simulink model "Two_Attitude_Estimation_ekf"  (R2021a)
settings: Solver=FixedStepAuto  StartTime=0.0  StopTime=200  FixedStep=Ts  RelTol=1e-5
values from neighbouring files (symbols this model uses):
  accel_filter_coef = [    0.0264    0.1405    0.3331    0.3331    0.1405    0.0264]    [quad_params_ekf.m]
  g = ref_acc(3)    [ekf_measurement_jacobian.m]    (also in quad_params_ekf.m = 9.81)
  gyro_filter_den = [ 1.0000    2.2287    2.5245    1.5773    0.5410    0.0796]    [quad_params_ekf.m]
  gyro_filter_num = [ 0.2821    1.2725    2.4208    2.4208    1.2725    0.2821]    [quad_params_ekf.m]
  I = [     0.005831943165131                   0                   0 ... (first row only)    [quad_params_ekf.m]
  Kd_rates = [0.05,0.05,0.1]'    [quad_params_ekf.m]
  Kd_vel = [0.8,0.8,0.3]'    [quad_params_ekf.m]
  Ki_vel = [0.1,0.1,0.1]'    [quad_params_ekf.m]
  km = 1.2e-7    (= 1.2e-07)    [quad_params_ekf.m]
  Kp_att = [6,6,6]'    [quad_params_ekf.m]
  Kp_pos = [7,7,3]'    [quad_params_ekf.m]
  Kp_rates = [10,10,10]'    [quad_params_ekf.m]
  Kp_vel = [3,3,5]'    [quad_params_ekf.m]
  kt = 0.9e-5    (= 9e-06)    [quad_params_ekf.m]
  L = 0.2    [quad_params_ekf.m]
  m = 0.9272    [quad_params_ekf.m]
  P_init = 0.01*eye(7)    [quad_params_ekf.m]
  Q = diag([0.015,0.0150,0.0150,0.0150,0.001,0.001,0.001])    [quad_params_ekf.m]
  q_init = [1;0;0;0]    [quad_params_ekf.m]
  R = diag([0.35,0.35,0.35,0.05,0.05,0.05])    [quad_params_ekf.m]
  rate_p_max = 3.5    [quad_params_ekf.m]
  thrust_max = thrust_max_per_motor*4    (= 32)    [quad_params_ekf.m]
  thrust_max_per_motor = 8    [quad_params_ekf.m]
  tilt_max = pi/6    (= 0.523598775598)    [quad_params_ekf.m]
  TQ_max_per_motor = km*(w_max.^2)    [quad_params_ekf.m]
  Ts = 0.001    [ekf_process_jacobian.m]    (also in ekf_process_model.m; quad_params_ekf.m)
  Ts_IMU = 0.001    [quad_params_ekf.m]
  Vb_init = [0;0;0]    [quad_params_ekf.m]
  vel_xy_max = 15    [quad_params_ekf.m]
  vel_z_max = 10    [quad_params_ekf.m]
  wb_init = [0;0;0]    [quad_params_ekf.m]
  x_0 = [1 0 0 0 0 0 0]'    [quad_params_ekf.m]
  Xe_init = [0;0;0]    [quad_params_ekf.m]
undefined symbols (not defined in the file or in its folder): IMU, p, pm_0, sigbuilder_block, Vm_0, xme_0
libraries: aerolibutil x8, simulink_extras x8, sharedtransform x7, sharedutil x6, simulink x4, pid_lib x3, aerolibcommonsys x3, aerolibnavsys x2, dspstat3 x2, mspsensorlib x1, aerolibnav x1, dspmtrx3 x1
(part 1 of 4)
settings Model: Creator=Petronas-Tareq  LastModifiedBy=Petronas-Tareq
settings SolverCC: AutoInsertRateTranBlk=on  InsertRTBMode=Always

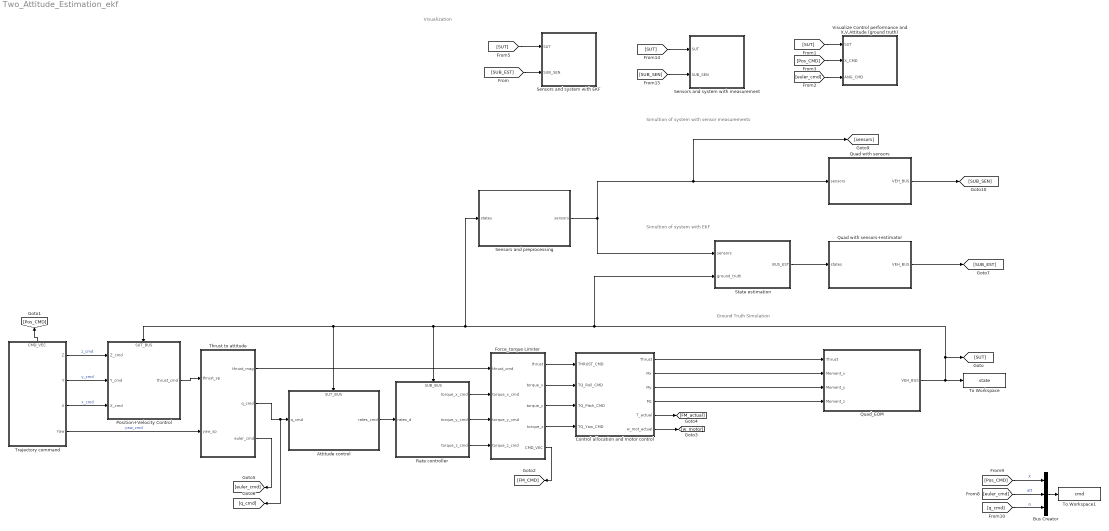
== system Two_Attitude_Estimation_ekf ==
  note: Simultion of system with sensor measurements
  note: Visualization
  note: Ground Truth Simulation
  note: Simultion of system with EKF
  Attitude control : Subsystem
      settings: PortSchema="{\"entries\":[{\"content\":{\"sides\":[{\"content\":{\"connectorIds\":[\"In1\"]},\"type\":\"ConnectorPlacement.EquallySpacedRectSide\",\"uuid\":\"19a574f6-5314-4727-8968-5b1c9712010e\"},{\"content\":{\"connectorIds\":[\"Out1\"],\"side\":\"RIGHT\"},\"type\":\"ConnectorPlacement.EquallySpacedRectSide\",\"uuid\":\"5cd6813f-6e17-48c1-918b-7c366c6d9cfa\"},{\"content\":{\"connectorIds\":[\"In2\"],\"side\":\"TOP\"},\"type\":\"ConnectorPlacement.EquallySpacedRectSide\",\"uuid\":\"b2bca67c-c4f4-4722-89a0-a16251073bfd\"}]},\"type\":\"ConnectorPlacement.EquallySpacedConnector\",\"uuid\":\"dcbf54f5-c136-40d5-a3db-9d2776e5196c\"}],\"packageUris\":[\"http://schema.mathworks.com/mf0/Connector/R2020b\"],\"version\":\"1.0\"}"
      mask Display: image('$imagefile'); % Use "Edit Image" on toolstrip to change.
  Bus Creator : BusCreator  Inputs=3
  Control allocation and motor control : Subsystem  Variant=on  VariantControlMode=label  LabelModeActiveChoice=Choice1
      mask Display: image('$imagefile'); % Use "Edit Image" on toolstrip to change.
  Force_torque Limiter : Subsystem
  Position+Velocity Control : Subsystem
      settings: PortSchema="{\"entries\":[{\"content\":{\"sides\":[{\"content\":{\"connectorIds\":[\"In1\",\"In2\",\"In3\"]},\"type\":\"ConnectorPlacement.EquallySpacedRectSide\",\"uuid\":\"cfe37ea9-b8e2-443a-9d65-596f0fda79c9\"},{\"content\":{\"connectorIds\":[\"Out1\"],\"side\":\"RIGHT\"},\"type\":\"ConnectorPlacement.EquallySpacedRectSide\",\"uuid\":\"f39f64e1-4b16-444a-b7d2-95ecb1b2a6fa\"},{\"content\":{\"connectorIds\":[\"In4\"],\"side\":\"TOP\"},\"type\":\"ConnectorPlacement.EquallySpacedRectSide\",\"uuid\":\"52402c3a-f2ac-44cf-8c94-dbfc3f851d2b\"}]},\"type\":\"ConnectorPlacement.EquallySpacedConnector\",\"uuid\":\"0122f56a-2702-493b-af7d-a25e6b9e04ed\"}],\"packageUris\":[\"http://schema.mathworks.com/mf0/Connector/R2020b\"],\"version\":\"1.0\"}"
  Quad with sensors : Subsystem
      mask Display: image('$imagefile'); % Use "Edit Image" on toolstrip to change.
  Quad with sensors+estimator : Subsystem
      mask Display: image('$imagefile'); % Use "Edit Image" on toolstrip to change.
  Quad_EOM : Subsystem
      mask Display: image('$imagefile'); % Use "Edit Image" on toolstrip to change.
  Rate controller : Subsystem
      settings: PortSchema="{\"entries\":[{\"content\":{\"sides\":[{\"content\":{\"connectorIds\":[\"In1\"]},\"type\":\"ConnectorPlacement.EquallySpacedRectSide\",\"uuid\":\"0af60e35-7b10-4750-a6af-1a3d920b4771\"},{\"content\":{\"connectorIds\":[\"Out1\",\"Out2\",\"Out3\"],\"side\":\"RIGHT\"},\"type\":\"ConnectorPlacement.EquallySpacedRectSide\",\"uuid\":\"931b0f34-b3f1-4a41-949f-3d763eca3151\"},{\"content\":{\"connectorIds\":[\"In2\"],\"side\":\"TOP\"},\"type\":\"ConnectorPlacement.EquallySpacedRectSide\",\"uuid\":\"84fe42fa-07d1-4fd9-ad2f-8c6651eaa98c\"}]},\"type\":\"ConnectorPlacement.EquallySpacedConnector\",\"uuid\":\"f603d2ac-5c20-4a82-ba8b-1c7971d6778a\"}],\"packageUris\":[\"http://schema.mathworks.com/mf0/Connector/R2020b\"],\"version\":\"1.0\"}"
  Sensors and preprocessing : Subsystem
  Sensors and system with EKF : Subsystem
  Sensors and system with measurement : Subsystem
  State estimation : Subsystem
  Thrust to attitude : Subsystem
  To Workspace : ToWorkspace  VariableName=state  SaveFormat=Timeseries  SampleTime=-1
  To Workspace1 : ToWorkspace  VariableName=cmd  SaveFormat=Timeseries  SampleTime=-1
  Trajectory command : Subsystem  Variant=on  VariantControlMode=label  LabelModeActiveChoice=5
      settings: PortSchema="{\"entries\":[{\"content\":{\"sides\":[{\"content\":{\"connectorIds\":[]},\"type\":\"ConnectorPlacement.EquallySpacedRectSide\",\"uuid\":\"8b658e99-682c-4d99-9859-63a6cdcf875c\"},{\"content\":{\"connectorIds\":[\"Out1\",\"Out2\",\"Out3\",\"Out4\"],\"side\":\"RIGHT\"},\"type\":\"ConnectorPlacement.EquallySpacedRectSide\",\"uuid\":\"566e7e32-52b1-45cc-9bb3-5343461c1cc0\"},{\"content\":{\"connectorIds\":[\"Out5\"],\"side\":\"TOP\"},\"type\":\"ConnectorPlacement.EquallySpacedRectSide\",\"uuid\":\"4cb1ab19-6483-4408-b5f4-106b35038f17\"}]},\"type\":\"ConnectorPlacement.EquallySpacedConnector\",\"uuid\":\"dc7c82fc-432d-4c18-9829-e6c2b483f5a7\"}],\"packageUris\":[\"http://schema.mathworks.com/mf0/Connector/R2020b\"],\"version\":\"1.0\"}"
  Visualize Control performance and X,V,Attitude (ground truth) : Subsystem
  wires:
  Force_torque Limiter/5(CMD_VEC) -> [FM_CMD]
  Trajectory command/2(Y) -> Position+Velocity Control/2(Y_cmd)  "y_cmd"
  Trajectory command/3(X) -> Position+Velocity Control/3(X_cmd)  "x_cmd"
  Control allocation and motor control/1(Thrust) -> Quad_EOM/1(Thrust)
  Control allocation and motor control/2(Mx) -> Quad_EOM/2(Moment_x)
  Control allocation and motor control/3(My) -> Quad_EOM/3(Moment_y)
  Control allocation and motor control/4(Mz) -> Quad_EOM/4(Moment_z)
  Control allocation and motor control/5(T_actual) -> [FM_actual]
  Control allocation and motor control/6(w_mot_actual) -> [w_motor]
  Trajectory command/1(Z) -> Position+Velocity Control/1(Z_cmd)  "z_cmd"
  Force_torque Limiter/4(torque_z) -> Control allocation and motor control/4(TQ_Yaw_CMD)
  Force_torque Limiter/3(torque_y) -> Control allocation and motor control/3(TQ_Pitch_CMD)
  Force_torque Limiter/2(torque_x) -> Control allocation and motor control/2(TQ_Roll_CMD)
  Force_torque Limiter/1(thrust) -> Control allocation and motor control/1(THRUST_CMD)
  Thrust to attitude/1(thrust_mag) -> Force_torque Limiter/1(thrust_cmd)
  Rate controller/2(torque_y_cmd) -> Force_torque Limiter/3(torque_y_cmd)
  Rate controller/3(torque_z_cmd) -> Force_torque Limiter/4(torque_z_cmd)
  Rate controller/1(torque_x_cmd) -> Force_torque Limiter/2(torque_x_cmd)
  Attitude control/1(rates_cmd) -> Rate controller/1(rates_d)
  Trajectory command/5(CMD_VEC) -> [Pos_CMD]
  Bus Creator/1 -> To Workspace1/1
  [Pos_CMD] -> Bus Creator/1  "X"
  [euler_cmd] -> Bus Creator/2  "att"
  [q_cmd] -> Bus Creator/3  "q"
  Thrust to attitude/2(q_cmd) -> Attitude control/1(q_cmd), [q_cmd]
  Thrust to attitude/3(euler_cmd) -> [euler_cmd]
  Trajectory command/4(Yaw) -> Thrust to attitude/2(yaw_sp)  "yaw_cmd"
  Position+Velocity Control/1(thrust_cmd) -> Thrust to attitude/1(thrust_sp)
  Quad_EOM/1(VEH_BUS) -> Sensors and preprocessing/1(states), Position+Velocity Control/4(SUT_BUS), Attitude control/2(SUT_BUS), Rate controller/2(SUB_BUS), State estimation/2(ground_truth), [SUT], To Workspace/1
  Sensors and preprocessing/1(sensors) -> Quad with sensors/1(sensors), [sensors], State estimation/1(sensors)
  Quad with sensors/1(VEH_BUS) -> [SUB_SEN]
  [SUB_SEN] -> Sensors and system with measurement/2(SUB_SEN)
  [SUT] -> Visualize Control performance and X,V,Attitude (ground truth)/1(SUT)
  [euler_cmd] -> Visualize Control performance and X,V,Attitude (ground truth)/3(ANG_CMD)
  [Pos_CMD] -> Visualize Control performance and X,V,Attitude (ground truth)/2(X_CMD)
  [SUT] -> Sensors and system with measurement/1(SUT)
  Quad with sensors+estimator/1(VEH_BUS) -> [SUB_EST]
  State estimation/1(BUS_EST) -> Quad with sensors+estimator/1(states)
  [SUT] -> Sensors and system with EKF/1(SUT)
  [SUB_EST] -> Sensors and system with EKF/2(SUB_SEN)

== system Two_Attitude_Estimation_ekf/Attitude control ==
  note: Attitude control (full attitude control, i.e. yaw+thrust)
  note: Attitude Error Calculation
  q_cmd : Inport
  SUT_BUS : Inport  Port=2
  Bus Selector3 : BusSelector  OutputSignals=q
  K_attitude : Gain  Gain=Kp_att
  MATLAB Function1 : MATLAB Function  TreatAsAtomicUnit=on
  Product : Product
  Quaternion Inverse : aerolibutil/Quaternion Inverse
  Quaternion multiply : aerolibutil/Quaternion Multiplication
  Selector1 : Selector  InputPortWidth=4  IndexOptions=Index vector (dialog)  Indices=1  OutputSizes=1
  Selector2 : Selector  InputPortWidth=4  IndexOptions=Index vector (dialog)  Indices=2:4  OutputSizes=1
  k : Gain  Gain=2
  rates_cmd : Outport  VectorParamsAs1DForOutWhenUnconnected=off
  wires:
  SUT_BUS/1 -> [SUT]
  q_cmd/1 -> Quaternion multiply/2  "q_d"
  [SUT] -> Bus Selector3/1
  Bus Selector3/1 -> Quaternion Inverse/1  "<q>"
  Product/1 -> k/1  "error"
  Selector1/1 -> MATLAB Function1/1(q0)  "q0"
  MATLAB Function1/1(y) -> Product/1
  Selector2/1 -> Product/2  "q_vec"
  Quaternion multiply/1 -> Selector2/1, Selector1/1  "qe"
  k/1 -> K_attitude/1
  Quaternion Inverse/1 -> Quaternion multiply/1
  K_attitude/1 -> rates_cmd/1  "rates_cmd"

== system Two_Attitude_Estimation_ekf/Control allocation and motor control ==
  note: 1) Add Subsystem or Model blocks as valid variant choices.
      | 2) You cannot connect blocks at this level. At simulation, connectivity is automatically
      | determined, based on the active variant and port name matching.
  THRUST_CMD : Inport
  TQ_Roll_CMD : Inport  Port=2
  TQ_Pitch_CMD : Inport  Port=3
  TQ_Yaw_CMD : Inport  Port=4
  Ideal Actuators with allocation : Subsystem  VariantControl=Choice2
  Ideal Actuattion (direct transfer) : Subsystem  VariantControl=Choice1
  Thrust : Outport
  Mx : Outport  Port=2
  My : Outport  Port=3
  Mz : Outport  Port=4
  T_actual : Outport  Port=5
  w_mot_actual : Outport  Port=6

== system Two_Attitude_Estimation_ekf/Force_torque Limiter ==
  thrust_cmd : Inport
  torque_x_cmd : Inport  Port=2
  torque_y_cmd : Inport  Port=3
  torque_z_cmd : Inport  Port=4
  Mux : Mux
  Saturation : Saturate  UpperLimit=thrust_max  LowerLimit=-thrust_max
      settings: AttributesFormatString=|
      | MAX =    %<UpperLimit>
      | MIN = %<LowerLimit>
  Saturation1 : Saturate  UpperLimit=2*TQ_max_per_motor  LowerLimit=-2*TQ_max_per_motor
      settings: AttributesFormatString=|
      | MAX =    %<UpperLimit>
      | MIN = %<LowerLimit>
  Saturation2 : Saturate  UpperLimit=thrust_max_per_motor*L  LowerLimit=-thrust_max_per_motor *L
      settings: AttributesFormatString=|
      | MAX =    %<UpperLimit>
      | MIN = %<LowerLimit>
  Saturation3 : Saturate  UpperLimit=thrust_max_per_motor*L  LowerLimit=-thrust_max_per_motor *L
      settings: AttributesFormatString=|
      | MAX =    %<UpperLimit>
      | MIN = %<LowerLimit>
  Scope : Scope
  thrust : Outport  VectorParamsAs1DForOutWhenUnconnected=off
  torque_x : Outport  Port=2  VectorParamsAs1DForOutWhenUnconnected=off
  torque_y : Outport  Port=3  VectorParamsAs1DForOutWhenUnconnected=off
  torque_z : Outport  Port=4  VectorParamsAs1DForOutWhenUnconnected=off
  CMD_VEC : Outport  Port=5  VectorParamsAs1DForOutWhenUnconnected=off
  wires:
  torque_z_cmd/1 -> Saturation1/1
  thrust_cmd/1 -> Saturation/1
  torque_y_cmd/1 -> Saturation2/1
  torque_x_cmd/1 -> Saturation3/1
  Saturation/1 -> [THRUST], thrust/1
  Saturation3/1 -> [TQ_Roll_X], torque_x/1
  Saturation2/1 -> [TQ_Pitch_Y], torque_y/1
  Saturation1/1 -> [TQ_Yaw_Z], torque_z/1
  Mux/1 -> Scope/1, CMD_VEC/1
  [THRUST] -> Mux/1
  [TQ_Roll_X] -> Mux/2
  [TQ_Pitch_Y] -> Mux/3
  [TQ_Yaw_Z] -> Mux/4

== system Two_Attitude_Estimation_ekf/Position+Velocity Control ==
  note: Velocity PID controller
  note: Position P controller
  Z_cmd : Inport
  Y_cmd : Inport  Port=2
  X_cmd : Inport  Port=3
  SUT_BUS : Inport  Port=4
  Bus Selector3 : BusSelector  OutputSignals=Xe,Ve
  Mux : Mux  Inputs=3
  Position P Controller : Subsystem
  To Workspace2 : ToWorkspace  VariableName=thrust_sp  SaveFormat=Timeseries  SampleTime=-1
  Velocity PID Controller : Subsystem
  acc setpoint : Constant  Value=[0;0;0]
  thrust_cmd : Outport
  wires:
  SUT_BUS/1 -> [SUT]
  [SUT] -> Bus Selector3/1
  Bus Selector3/1 -> [P]  "<Xe>"
  Mux/1 -> [P_sp]
  acc setpoint/1 -> [acc_sp]
  [acc_sp] -> Velocity PID Controller/3(acc_ff)  "acc_feedforwad"
  Position P Controller/1(V_sp) -> Velocity PID Controller/1(vel_cmd)  "vel_cmd"
  [P_sp] -> Position P Controller/1(pos_cmd)
  [P] -> Position P Controller/2(pos_cur)
  [V] -> Velocity PID Controller/2(vel_cur)
  Velocity PID Controller/1(thrust_sp) -> To Workspace2/1, thrust_cmd/1  "thrust_cmd"
  Bus Selector3/2 -> [V]  "<Ve>"
  Z_cmd/1 -> Mux/3
  X_cmd/1 -> Mux/1
  Y_cmd/1 -> Mux/2

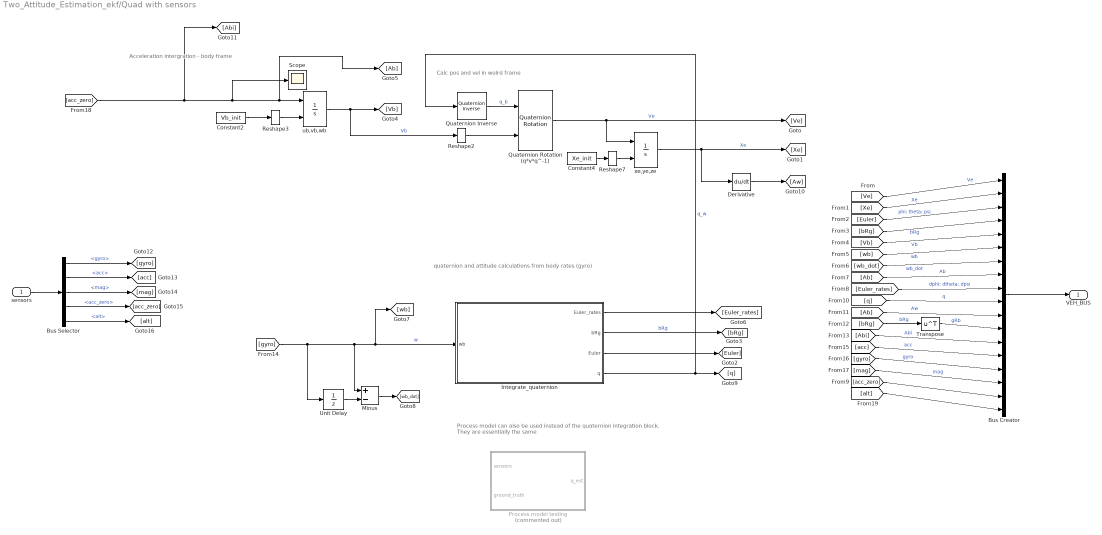
== system Two_Attitude_Estimation_ekf/Quad with sensors ==
  note: Process model can also be used instead of the
      |  quaternion integration block. They are essentially the same
  note: Acceleration intergration - body frame
  note: Calc pos and vel in wolrd frame
  note: quaternion and attitude calculations from body rates (gyro)
  sensors : Inport
  Bus Creator : BusCreator  Inputs=18
  Bus Selector : BusSelector  OutputSignals=gyro,acc,mag,acc_zero,alt
  Constant2 : Constant  Value=Vb_init  OutDataTypeStr=Inherit: Inherit via back propagation
  Constant4 : Constant  Value=Xe_init  OutDataTypeStr=Inherit: Inherit via back propagation
  Derivative : Derivative
  Integrate_quaternion : Subsystem
  Minus : Sum  Inputs=+-
  Process model testing : Subsystem  Commented=on
  Quaternion Inverse : aerolibutil/Quaternion Inverse
  Quaternion Rotation (q*v*q^-1) : aerolibutil/Quaternion Rotation
  Reshape2 : Reshape  OutputDimensionality=Column vector (2-D)
  Reshape3 : Reshape  OutputDimensionality=Column vector (2-D)
  Reshape7 : Reshape  OutputDimensionality=Column vector (2-D)
  Scope : Scope
  Transpose : Math  Operator=transpose  SaturateOnIntegerOverflow=on
  Unit Delay : UnitDelay  SampleTime=-1  HasFrameUpgradeWarning=on
  ub,vb,wb : Integrator  InitialConditionSource=external  InitialCondition=Vm_0
  xe,ye,ze : Integrator  InitialConditionSource=external  InitialCondition=xme_0
  VEH_BUS : Outport  VectorParamsAs1DForOutWhenUnconnected=off
  wires:
  [Euler] -> Bus Creator/3  "phi; theta; psi"
  [Xe] -> Bus Creator/2  "Xe"
  [Ve] -> Bus Creator/1  "Ve"
  [bRg] -> Bus Creator/4  "bRg"
  [Ab] -> Bus Creator/8  "Ab"
  [wb_dot] -> Bus Creator/7  "wb_dot"
  Bus Creator/1 -> VEH_BUS/1
  [Vb] -> Bus Creator/5  "Vb"
  [wb] -> Bus Creator/6  "wb"
  [Euler_rates] -> Bus Creator/9  "dphi; dtheta; dpsi"
  Constant2/1 -> Reshape3/1
  Integrate_quaternion/2(bRg) -> [bRg]  "bRg"
  Constant4/1 -> Reshape7/1
  Reshape3/1 -> ub,vb,wb/2
  Reshape7/1 -> xe,ye,ze/2
  Quaternion Rotation (q*v*q^-1)/1 -> xe,ye,ze/1, [Ve]  "Ve"
  xe,ye,ze/1 -> Derivative/1, [Xe]  "Xe"
  [gyro] -> Unit Delay/1, Minus/1, Integrate_quaternion/1(wb), [wb]  "w"
  ub,vb,wb/1 -> [Vb], Reshape2/1  "Vb"
  Integrate_quaternion/1(Euler_rates) -> [Euler_rates]
  Integrate_quaternion/3(Euler) -> [Euler]
  [q] -> Bus Creator/10  "q"
  Integrate_quaternion/4(q) -> Quaternion Inverse/1, [q]  "q_w"
  Reshape2/1 -> Quaternion Rotation (q*v*q^-1)/2
  Quaternion Inverse/1 -> Quaternion Rotation (q*v*q^-1)/1  "q_b"
  Derivative/1 -> [Aw]
  [Ab] -> Bus Creator/11  "Aw"
  [bRg] -> Transpose/1  "bRg"
  Transpose/1 -> Bus Creator/12  "gRb"
  [Abi] -> Bus Creator/13  "Abi"
  Unit Delay/1 -> Minus/2
  Minus/1 -> [wb_dot]
  Bus Selector/1 -> [gyro]  "<gyro>"
  Bus Selector/2 -> [acc]  "<acc>"
  sensors/1 -> Bus Selector/1
  [acc_zero] -> [Abi], Scope/1, [Ab], ub,vb,wb/1
  [acc] -> Bus Creator/14  "acc"
  [gyro] -> Bus Creator/15  "gyro"
  Bus Selector/3 -> [mag]  "<mag>"
  [mag] -> Bus Creator/16  "mag"
  Bus Selector/4 -> [acc_zero]  "<acc_zero>"
  [acc_zero] -> Bus Creator/17
  Bus Selector/5 -> [alt]  "<alt>"
  [alt] -> Bus Creator/18

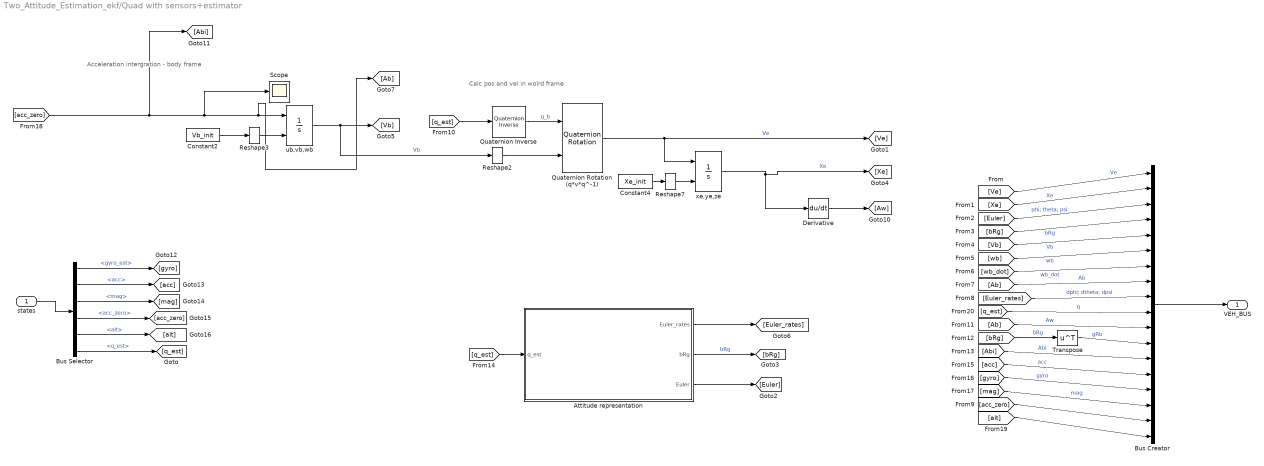
== system Two_Attitude_Estimation_ekf/Quad with sensors+estimator ==
  note: Calc pos and vel in wolrd frame
  note: Acceleration intergration - body frame
  states : Inport
  Attitude representation : Subsystem
  Bus Creator : BusCreator  Inputs=18
  Bus Selector : BusSelector  OutputSignals=gyro_est,acc,mag,acc_zero,alt,q_est
  Constant2 : Constant  Value=Vb_init  OutDataTypeStr=Inherit: Inherit via back propagation
  Constant4 : Constant  Value=Xe_init  OutDataTypeStr=Inherit: Inherit via back propagation
  Derivative : Derivative
  Quaternion Inverse : aerolibutil/Quaternion Inverse
  Quaternion Rotation (q*v*q^-1) : aerolibutil/Quaternion Rotation
  Reshape2 : Reshape  OutputDimensionality=Column vector (2-D)
  Reshape3 : Reshape  OutputDimensionality=Column vector (2-D)
  Reshape7 : Reshape  OutputDimensionality=Column vector (2-D)
  Scope : Scope
  Transpose : Math  Operator=transpose  SaturateOnIntegerOverflow=on
  ub,vb,wb : Integrator  InitialConditionSource=external  InitialCondition=Vm_0
  xe,ye,ze : Integrator  InitialConditionSource=external  InitialCondition=xme_0
  VEH_BUS : Outport  VectorParamsAs1DForOutWhenUnconnected=off
  wires:
  [Euler] -> Bus Creator/3  "phi; theta; psi"
  [Xe] -> Bus Creator/2  "Xe"
  [Ve] -> Bus Creator/1  "Ve"
  [bRg] -> Bus Creator/4  "bRg"
  [Ab] -> Bus Creator/8  "Ab"
  [wb_dot] -> Bus Creator/7  "wb_dot"
  Bus Creator/1 -> VEH_BUS/1
  [Vb] -> Bus Creator/5  "Vb"
  [wb] -> Bus Creator/6  "wb"
  [Euler_rates] -> Bus Creator/9  "dphi; dtheta; dpsi"
  Attitude representation/2(bRg) -> [bRg]  "bRg"
  Attitude representation/1(Euler_rates) -> [Euler_rates]
  Attitude representation/3(Euler) -> [Euler]
  [q_est] -> Bus Creator/10  "q"
  [Ab] -> Bus Creator/11  "Aw"
  [bRg] -> Transpose/1  "bRg"
  Transpose/1 -> Bus Creator/12  "gRb"
  [Abi] -> Bus Creator/13  "Abi"
  Bus Selector/1 -> [gyro]  "<gyro_est>"
  Bus Selector/2 -> [acc]  "<acc>"
  states/1 -> Bus Selector/1
  [acc] -> Bus Creator/14  "acc"
  [gyro] -> Bus Creator/15  "gyro"
  Bus Selector/3 -> [mag]  "<mag>"
  [mag] -> Bus Creator/16  "mag"
  Bus Selector/4 -> [acc_zero]  "<acc_zero>"
  [acc_zero] -> Bus Creator/17
  [alt] -> Bus Creator/18
  [q_est] -> Attitude representation/1(q_est)
  Bus Selector/5 -> [alt]  "<alt>"
  Bus Selector/6 -> [q_est]  "<q_est>"
  Quaternion Rotation (q*v*q^-1)/1 -> xe,ye,ze/1, [Ve]  "Ve"
  [acc_zero] -> [Abi], Scope/1, [Ab], ub,vb,wb/1
  ub,vb,wb/1 -> [Vb], Reshape2/1  "Vb"
  Constant4/1 -> Reshape7/1
  Derivative/1 -> [Aw]
  xe,ye,ze/1 -> Derivative/1, [Xe]  "Xe"
  Reshape2/1 -> Quaternion Rotation (q*v*q^-1)/2
  Reshape7/1 -> xe,ye,ze/2
  Reshape3/1 -> ub,vb,wb/2
  Quaternion Inverse/1 -> Quaternion Rotation (q*v*q^-1)/1  "q_b"
  Constant2/1 -> Reshape3/1
  [q_est] -> Quaternion Inverse/1

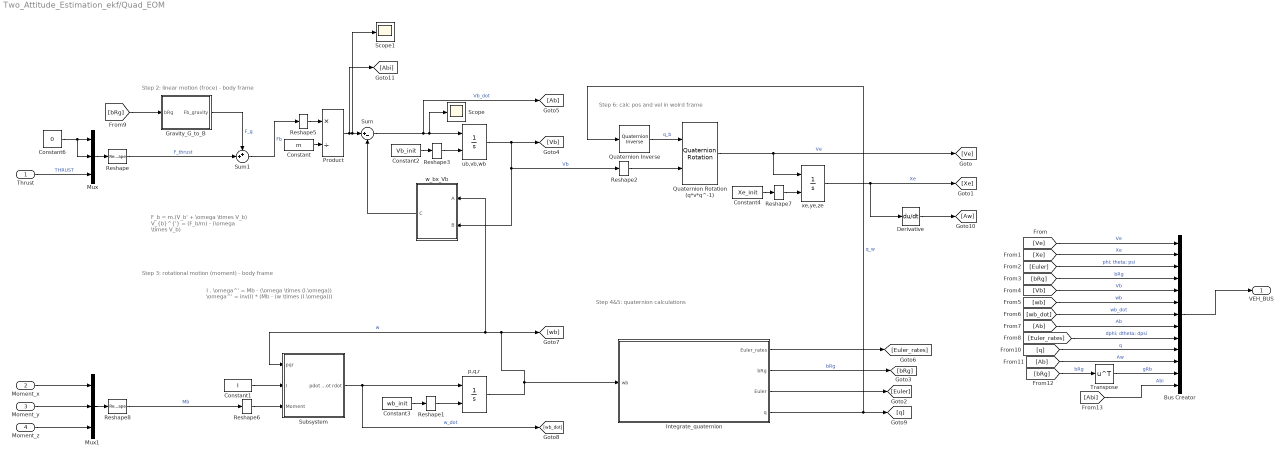
== system Two_Attitude_Estimation_ekf/Quad_EOM ==
  note: Step 3: rotational motion (moment) - body frame
  note: F_b = m.(V_b' + \omega \times V_b)
      |
      | V_{b}^{'} = (F_b/m) - (\omega \times V_b)
  note: Step 2: linear motion (froce) - body frame
  note: Step 6: calc pos and vel in wolrd frame
  note: I . \omega^' = Mb - (\omega \times (I.\omega))
      |
      | \omega^' = inv(I) * (Mb - (w \times (I.\omega)))
  note: Step 4&5: quaternion calculations
  Thrust : Inport
  Moment_x : Inport  Port=2
  Moment_y : Inport  Port=3
  Moment_z : Inport  Port=4
  Bus Creator : BusCreator  Inputs=13
  Constant : Constant  Value=m  OutDataTypeStr=Inherit: Inherit via back propagation
  Constant1 : Constant  Value=I  OutDataTypeStr=Inherit: Inherit via back propagation
  Constant2 : Constant  Value=Vb_init  OutDataTypeStr=Inherit: Inherit via back propagation
  Constant3 : Constant  Value=wb_init  OutDataTypeStr=Inherit: Inherit via back propagation
  Constant4 : Constant  Value=Xe_init  OutDataTypeStr=Inherit: Inherit via back propagation
  Constant6 : Constant  Value=0
  Derivative : Derivative
  Gravity_G_to_B : Subsystem
  Integrate_quaternion : Subsystem
  Mux : Mux  Inputs=3
  Mux1 : Mux  Inputs=3
  Product : Product  Inputs=*/  SaturateOnIntegerOverflow=on  OutDataTypeStr=Inherit: Same as first input
  Quaternion Inverse : aerolibutil/Quaternion Inverse
  Quaternion Rotation (q*v*q^-1) : aerolibutil/Quaternion Rotation
  Reshape{,1..3,5..8} (8 alike) : Reshape  OutputDimensionality=Column vector (2-D)
  Scope : Scope
  Scope1 : Scope
  Subsystem : Subsystem
  Sum : Sum  Inputs=|+-  SaturateOnIntegerOverflow=on
  Sum1 : Sum  Inputs=++|
  Transpose : Math  Operator=transpose  SaturateOnIntegerOverflow=on
  "p,q,r " : Integrator  InitialConditionSource=external  InitialCondition=pm_0
  ub,vb,wb : Integrator  InitialConditionSource=external  InitialCondition=Vm_0
  w_bx_Vb : Subsystem
      mask Display:
      | text(.5,.5,'Cross\nProduct\n\nC = AxB', ...
      | 	'HorizontalAlignment','Center',...
      | 	'VerticalAlignment','middle')
  xe,ye,ze : Integrator  InitialConditionSource=external  InitialCondition=xme_0
  VEH_BUS : Outport  VectorParamsAs1DForOutWhenUnconnected=off
  wires:
  [Euler] -> Bus Creator/3  "phi; theta; psi"
  [Xe] -> Bus Creator/2  "Xe"
  [Ve] -> Bus Creator/1  "Ve"
  [bRg] -> Bus Creator/4  "bRg"
  [Ab] -> Bus Creator/8  "Ab"
  [wb_dot] -> Bus Creator/7  "wb_dot"
  Bus Creator/1 -> VEH_BUS/1
  [Vb] -> Bus Creator/5  "Vb"
  [wb] -> Bus Creator/6  "wb"
  [Euler_rates] -> Bus Creator/9  "dphi; dtheta; dpsi"
  Reshape8/1 -> Reshape6/1  "Mb"
  Reshape6/1 -> Subsystem/3(Moment)
  Reshape1/1 -> "p,q,r "/2
  Constant2/1 -> Reshape3/1
  Subsystem/1(pdot qdot rdot) -> [wb_dot], "p,q,r "/1  "w_dot"
  Constant/1 -> Product/2
  Constant1/1 -> Subsystem/2(I)
  w_bx_Vb/1(C) -> Sum/2
  Integrate_quaternion/2(bRg) -> [bRg]  "bRg"
  Sum/1 -> [Ab], Scope/1, ub,vb,wb/1  "Vb_dot"
  Constant4/1 -> Reshape7/1
  Reshape3/1 -> ub,vb,wb/2
  Reshape7/1 -> xe,ye,ze/2
  Quaternion Rotation (q*v*q^-1)/1 -> xe,ye,ze/1, [Ve]  "Ve"
  Reshape5/1 -> Product/1
  xe,ye,ze/1 -> Derivative/1, [Xe]  "Xe"
  Sum1/1 -> Reshape5/1  "Fb"
  Constant3/1 -> Reshape1/1
  Product/1 -> [Abi], Scope1/1, Sum/1
  Constant6/1 -> Mux/2, Mux/1
  Gravity_G_to_B/1(Fb_gravity) -> Sum1/1  "F_g"
  Mux/1 -> Reshape/1
  Reshape/1 -> Sum1/2  "F_thrust"
  Thrust/1 -> Mux/3  "THRUST"
  [bRg] -> Gravity_G_to_B/1(bRg)
  Moment_y/1 -> Mux1/2
  Moment_z/1 -> Mux1/3
  Mux1/1 -> Reshape8/1
  Moment_x/1 -> Mux1/1
  "p,q,r "/1 -> [wb], Subsystem/1(pqr), w_bx_Vb/1(A), Integrate_quaternion/1(wb)  "w"
  ub,vb,wb/1 -> [Vb], Reshape2/1, w_bx_Vb/2(B)  "Vb"
  Integrate_quaternion/1(Euler_rates) -> [Euler_rates]
  Integrate_quaternion/3(Euler) -> [Euler]
  [q] -> Bus Creator/10  "q"
  Integrate_quaternion/4(q) -> Quaternion Inverse/1, [q]  "q_w"
  Reshape2/1 -> Quaternion Rotation (q*v*q^-1)/2
  Quaternion Inverse/1 -> Quaternion Rotation (q*v*q^-1)/1  "q_b"
  Derivative/1 -> [Aw]
  [Ab] -> Bus Creator/11  "Aw"
  [bRg] -> Transpose/1  "bRg"
  Transpose/1 -> Bus Creator/12  "gRb"
  [Abi] -> Bus Creator/13  "Abi"

== system Two_Attitude_Estimation_ekf/Rate controller ==
  note: Rate controller
  rates_d : Inport
  SUB_BUS : Inport  Port=2
  Bus Selector1 : BusSelector  OutputSignals=wb,wb_dot
  Demux : Demux  Outputs=3
  Kd_rates : Gain  Gain=Kd_rates
  Kp_rates : Gain  Gain=Kp_rates
  Scope : Scope  NumInputPorts=2
  Sum : Sum  Inputs=|+-
  Sum1 : Sum  Inputs=|+-
  limit rate p : Saturate  UpperLimit=rate_p_max  LowerLimit=-rate_p_max
  limit rate q : Saturate  UpperLimit=rate_p_max  LowerLimit=-rate_p_max
  limit rate r : Saturate  UpperLimit=rate_p_max  LowerLimit=-rate_p_max
  torque_x_cmd : Outport
  torque_y_cmd : Outport  Port=2
  torque_z_cmd : Outport  Port=3
  wires:
  Bus Selector1/2 -> Kd_rates/1  "<wb_dot>"
  Bus Selector1/1 -> Sum1/2, Scope/2  "<wb>"
  Demux/1 -> limit rate p/1
  Demux/2 -> limit rate q/1
  Demux/3 -> limit rate r/1
  SUB_BUS/1 -> Bus Selector1/1  "measurements"
  rates_d/1 -> Sum1/1, Scope/1
  Kd_rates/1 -> Sum/2  "w_d"
  Kp_rates/1 -> Sum/1
  Sum/1 -> Demux/1  "torques"
  Sum1/1 -> Kp_rates/1
  limit rate p/1 -> torque_x_cmd/1
  limit rate q/1 -> torque_y_cmd/1
  limit rate r/1 -> torque_z_cmd/1

== system Two_Attitude_Estimation_ekf/Sensors and preprocessing ==
  states : Inport
  Bus Creator4 : BusCreator  Inputs=5
  IMU+altitude : Subsystem
  Memory1 : Memory  InheritSampleTime=on
  Preprocessing and Filtering : Subsystem
  Scope : Scope
  Scope1 : Scope
  sensors : Outport
  wires:
  states/1 -> Memory1/1
  Bus Creator4/1 -> sensors/1
  IMU+altitude/1(acc) -> Scope/1, Preprocessing and Filtering/1(acc_raw)  "acc_raw"
  IMU+altitude/2(gyro) -> Scope1/1, Preprocessing and Filtering/2(gyro_raw)  "gyro_raw"
  Memory1/1 -> IMU+altitude/1(States)
  IMU+altitude/3(alt) -> Preprocessing and Filtering/3(alt_raw)  "alt_raw"
  IMU+altitude/4(mag) -> Preprocessing and Filtering/4(mag_raw)  "mag_raw"
  Preprocessing and Filtering/1(acc_zero) -> Bus Creator4/1  "acc_zero"
  Preprocessing and Filtering/2(acc) -> Bus Creator4/2  "acc"
  Preprocessing and Filtering/3(gyro) -> Bus Creator4/3  "gyro"
  Preprocessing and Filtering/4(alt) -> Bus Creator4/4  "alt"
  Preprocessing and Filtering/5(mag) -> Bus Creator4/5  "mag"

== system Two_Attitude_Estimation_ekf/Sensors and system with EKF ==
  note: Confirm sensors are simulated properly
  SUT : Inport
  SUB_SEN : Inport  Port=2
  "Attitude " : Scope  NumInputPorts=3
  Bus Selector : BusSelector  OutputSignals=wb
  Bus Selector1 : BusSelector  OutputSignals=phi; theta; psi
  Bus Selector2 : BusSelector  OutputSignals=Xe
  Bus Selector21 : BusSelector  OutputSignals=Xe
  Bus Selector3 : BusSelector  OutputSignals=Abi
  Bus Selector4 : BusSelector  OutputSignals=gyro
  Bus Selector5 : BusSelector  OutputSignals=acc_zero
  Bus Selector8 : BusSelector  OutputSignals=phi; theta; psi
  Demux{1..2,9,11} (4 alike) : Demux  Outputs=3
  Mux{,1..2,4..6} (6 alike) : Mux  Inputs=2
  Position : Scope  NumInputPorts=3
  Scope : Scope  NumInputPorts=2
  Scope1 : Scope  NumInputPorts=2
  wires:
  Mux4/1 -> Position/1
  Demux11/2 -> Mux5/1  "y"
  [SUT] -> Bus Selector21/1
  Demux11/1 -> Mux4/1  "x"
  Mux5/1 -> Position/2
  Demux11/3 -> Mux6/1  "z"
  Bus Selector21/1 -> Demux11/1  "<Xe>"
  [SUT] -> Bus Selector8/1
  Mux6/1 -> Position/3
  Bus Selector8/1 -> Demux9/1  "<phi; theta; psi>"
  Mux2/1 -> "Attitude "/3
  Demux9/2 -> Mux1/1  "pitch"
  Demux9/3 -> Mux2/1  "yaw"
  Mux1/1 -> "Attitude "/2
  Mux/1 -> "Attitude "/1
  Demux9/1 -> Mux/1  "roll"
  SUT/1 -> [SUT]
  SUB_SEN/1 -> [SUB_SEN]
  [SUB_SEN] -> Bus Selector1/1
  Bus Selector1/1 -> Demux1/1  "<phi; theta; psi>"
  Demux1/1 -> Mux/2  "roll_est"
  Demux1/2 -> Mux1/2  "pitch_est"
  Demux1/3 -> Mux2/2  "yaw_est"
  [SUB_SEN] -> Bus Selector2/1
  Bus Selector2/1 -> Demux2/1  "<Xe>"
  Demux2/1 -> Mux4/2  "x_est"
  Demux2/2 -> Mux5/2  "y_est"
  Demux2/3 -> Mux6/2  "z_est"
  Bus Selector/1 -> Scope/2  "<wb>"
  Bus Selector4/1 -> Scope/1  "<gyro>"
  Bus Selector5/1 -> Scope1/1  "<acc_zero>"
  [SUT] -> Bus Selector3/1
  [SUB_SEN] -> Bus Selector4/1
  [SUB_SEN] -> Bus Selector5/1
  [SUT] -> Bus Selector/1
  Bus Selector3/1 -> Scope1/2  "<Abi>"

== system Two_Attitude_Estimation_ekf/Sensors and system with measurement ==
  note: Confirm sensors are simulated properly
  SUT : Inport
  SUB_SEN : Inport  Port=2
  "Attitude " : Scope  NumInputPorts=3
  Bus Selector : BusSelector  OutputSignals=wb
  Bus Selector1 : BusSelector  OutputSignals=phi; theta; psi
  Bus Selector2 : BusSelector  OutputSignals=Xe
  Bus Selector21 : BusSelector  OutputSignals=Xe
  Bus Selector3 : BusSelector  OutputSignals=Abi
  Bus Selector4 : BusSelector  OutputSignals=gyro
  Bus Selector5 : BusSelector  OutputSignals=acc_zero
  Bus Selector8 : BusSelector  OutputSignals=phi; theta; psi
  Demux{1..2,9,11} (4 alike) : Demux  Outputs=3
  Mux{,1..2,4..6} (6 alike) : Mux  Inputs=2
  Position : Scope  NumInputPorts=3
  Scope : Scope  NumInputPorts=2
  Scope1 : Scope  NumInputPorts=2
  wires:
  Mux4/1 -> Position/1
  Demux11/2 -> Mux5/1  "y"
  [SUT] -> Bus Selector21/1
  Demux11/1 -> Mux4/1  "x"
  Mux5/1 -> Position/2
  Demux11/3 -> Mux6/1  "z"
  Bus Selector21/1 -> Demux11/1  "<Xe>"
  [SUT] -> Bus Selector8/1
  Mux6/1 -> Position/3
  Bus Selector8/1 -> Demux9/1  "<phi; theta; psi>"
  Mux2/1 -> "Attitude "/3
  Demux9/2 -> Mux1/1  "pitch"
  Demux9/3 -> Mux2/1  "yaw"
  Mux1/1 -> "Attitude "/2
  Mux/1 -> "Attitude "/1
  Demux9/1 -> Mux/1  "roll"
  SUT/1 -> [SUT]
  SUB_SEN/1 -> [SUB_SEN]
  [SUB_SEN] -> Bus Selector1/1
  Bus Selector1/1 -> Demux1/1  "<phi; theta; psi>"
  Demux1/1 -> Mux/2  "roll_est"
  Demux1/2 -> Mux1/2  "pitch_est"
  Demux1/3 -> Mux2/2  "yaw_est"
  [SUB_SEN] -> Bus Selector2/1
  Bus Selector2/1 -> Demux2/1  "<Xe>"
  Demux2/1 -> Mux4/2  "x_est"
  Demux2/2 -> Mux5/2  "y_est"
  Demux2/3 -> Mux6/2  "z_est"
  Bus Selector/1 -> Scope/2  "<wb>"
  Bus Selector4/1 -> Scope/1  "<gyro>"
  Bus Selector5/1 -> Scope1/1  "<acc_zero>"
  [SUT] -> Bus Selector3/1
  [SUB_SEN] -> Bus Selector4/1
  [SUB_SEN] -> Bus Selector5/1
  [SUT] -> Bus Selector/1
  Bus Selector3/1 -> Scope1/2  "<Abi>"

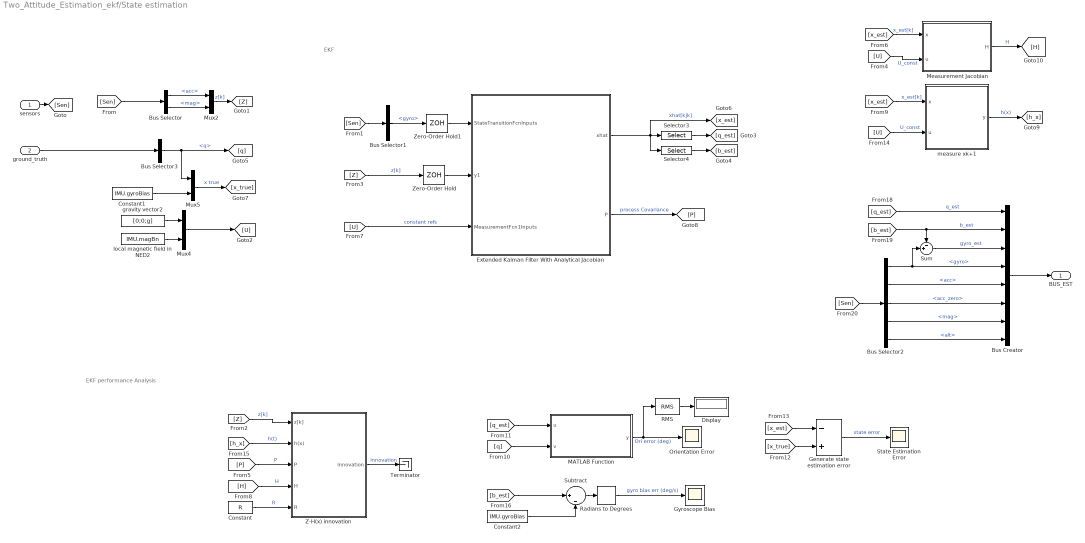
== system Two_Attitude_Estimation_ekf/State estimation ==
  note: EKF
  note: EKF performance Analysis
  sensors : Inport
  ground_truth : Inport  Port=2
  Bus Creator : BusCreator  Inputs=8
  Bus Selector : BusSelector  OutputSignals=acc,mag
  Bus Selector1 : BusSelector  OutputSignals=gyro
  Bus Selector2 : BusSelector  OutputSignals=gyro,acc,acc_zero,mag,alt
  Bus Selector3 : BusSelector  OutputSignals=q
  Constant : Constant  Value=R
  Constant1 : Constant  Value=IMU.gyroBias
  Constant2 : Constant  Value=IMU.gyroBias
  Display : Display
  Extended Kalman Filter With Analytical Jacobian : Subsystem  AncestorBlock=sharedTrackingLibrary/Extended Kalman Filter  mask(Extended Kalman Filter){StateTransitionFcn=ekf_process_model, HasStateTransitionJacobianFcn=on, StateTransitionJacobianFcn=ekf_process_jacobian, HasAdditiveProcessNoise=Additive, ProcessNoise=Q, HasTimeVaryingProcessNoise=off, HasStateTransitionFcnExtraArgument=1, InitialState=x_0, InitialStateCovariance=P_init, MeasurementFcn1=ekf_measurement_model, HasMeasurementJacobianFcn1=on, MeasurementJacobianFcn1=ekf_measurement_jacobian, HasMeasurementEnablePort1=off, HasAdditiveMeasurementNoise1=Additive, MeasurementNoise1=R, HasTimeVaryingMeasurementNoise1=off, HasMeasurementFcnExtraArgument1=1, MeasurementFcn2=myMeasurementFcn, HasMeasurementJacobianFcn2=off, MeasurementJacobianFcn2=, HasMeasurementEnablePort2=off, HasAdditiveMeasurementNoise2=Additive, MeasurementNoise2=1, HasTimeVaryingMeasurementNoise2=off, HasMeasurementFcnExtraArgument2=0, MeasurementFcn3=myMeasurementFcn, HasMeasurementJacobianFcn3=off, MeasurementJacobianFcn3=, HasMeasurementEnablePort3=off, HasAdditiveMeasurementNoise3=Additive, MeasurementNoise3=1, HasTimeVaryingMeasurementNoise3=off, HasMeasurementFcnExtraArgument3=0, MeasurementFcn4=myMeasurementFcn, HasMeasurementJacobianFcn4=off, MeasurementJacobianFcn4=, HasMeasurementEnablePort4=off, HasAdditiveMeasurementNoise4=Additive, MeasurementNoise4=1, HasTimeVaryingMeasurementNoise4=off, HasMeasurementFcnExtraArgument4=0, MeasurementFcn5=myMeasurementFcn, HasMeasurementJacobianFcn5=off, MeasurementJacobianFcn5=, HasMeasurementEnablePort5=off, HasAdditiveMeasurementNoise5=Additive, MeasurementNoise5=1, HasTimeVaryingMeasurementNoise5=off, HasMeasurementFcnExtraArgument5=0, EnableMultirate=off, StateTransitionFcnSampleTime=1, MeasurementFcn1SampleTime=1, MeasurementFcn2SampleTime=1, MeasurementFcn3SampleTime=1, MeasurementFcn4SampleTime=1, MeasurementFcn5SampleTime=1, UseCurrentEstimator=off, OutputStateCovariance=on, DataType=double, SampleTime=Ts, NumberOfMeasurements=1}
      mask prompts: HasStateTransitionJacobianFcn "shared_tracking:blocks:maskPromptEKFJacobian"; HasTimeVaryingProcessNoise "shared_tracking:blocks:maskPromptEKFUKFTimeVarying"; HasMeasurementJacobianFcn1 "shared_tracking:blocks:maskPromptEKFJacobian"; HasMeasurementEnablePort1 "shared_tracking:blocks:maskPromptEnablePort"; HasTimeVaryingMeasurementNoise1 "shared_tracking:blocks:maskPromptEKFUKFTimeVarying"; HasMeasurementJacobianFcn2 "shared_tracking:blocks:maskPromptEKFJacobian"; HasMeasurementEnablePort2 "shared_tracking:blocks:maskPromptEnablePort"; HasTimeVaryingMeasurementNoise2 "shared_tracking:blocks:maskPromptEKFUKFTimeVarying"; HasMeasurementJacobianFcn3 "shared_tracking:blocks:maskPromptEKFJacobian"; HasMeasurementEnablePort3 "shared_tracking:blocks:maskPromptEnablePort"; HasTimeVaryingMeasurementNoise3 "shared_tracking:blocks:maskPromptEKFUKFTimeVarying"; HasMeasurementJacobianFcn4 "shared_tracking:blocks:maskPromptEKFJacobian"; HasMeasurementEnablePort4 "shared_tracking:blocks:maskPromptEnablePort"; HasTimeVaryingMeasurementNoise4 "shared_tracking:blocks:maskPromptEKFUKFTimeVarying"; HasMeasurementJacobianFcn5 "shared_tracking:blocks:maskPromptEKFJacobian"; HasMeasurementEnablePort5 "shared_tracking:blocks:maskPromptEnablePort"; HasTimeVaryingMeasurementNoise5 "shared_tracking:blocks:maskPromptEKFUKFTimeVarying"; EnableMultirate "shared_tracking:blocks:maskPromptEnableMultirate"; StateTransitionFcnSampleTime "shared_tracking:blocks:maskPromptStateTransition"; MeasurementFcn1SampleTime "shared_tracking:blocks:maskPromptMeasurement1"; MeasurementFcn2SampleTime "shared_tracking:blocks:maskPromptMeasurement2"; MeasurementFcn3SampleTime "shared_tracking:blocks:maskPromptMeasurement3"; MeasurementFcn4SampleTime "shared_tracking:blocks:maskPromptMeasurement4"; MeasurementFcn5SampleTime "shared_tracking:blocks:maskPromptMeasurement5"; UseCurrentEstimator "shared_tracking:blocks:maskPromptUseCurrentEstimator"; OutputStateCovariance "shared_tracking:blocks:maskPromptOutputStateCovariance"; DataType "shared_tracking:blocks:maskPromptDataType"; SampleTime "shared_tracking:blocks:maskPromptSampleTime"
      mask help: shared_tracking:blocks:maskPromptEKFDescription
      mask init:
      | matlabshared.tracking.internal.blocks.maskInitializationScriptEKF
      mask Help: eval('matlabshared.tracking.internal.blocks.controlIdentLaunchDocPage(''EKF'')')
      mask Callback HasStateTransitionJacobianFcn: matlabshared.tracking.internal.blocks.dialogCallbacksEKFUKFPF(gcbh(),'checkBoxHasJacobianFcn','StateTransition');
      mask TypeOptions HasAdditiveProcessNoise: shared_tracking:blocks:maskPromptEKFUKFAdditiveNoise | shared_tracking:blocks:maskPromptEKFUKFNonAdditiveNoise
      mask Callback HasTimeVaryingProcessNoise: matlabshared.tracking.internal.blocks.dialogCallbacksEKFUKFPF(gcbh,'checkboxIsCovarianceTimeVarying','HasTimeVaryingProcessNoise','ProcessNoise')
      mask Callback HasMeasurementJacobianFcn1: matlabshared.tracking.internal.blocks.dialogCallbacksEKFUKFPF(gcbh(),'checkBoxHasJacobianFcn','Measurement','1');
      mask TypeOptions HasAdditiveMeasurementNoise1: shared_tracking:blocks:maskPromptEKFUKFAdditiveNoise | shared_tracking:blocks:maskPromptEKFUKFNonAdditiveNoise
      mask Callback HasTimeVaryingMeasurementNoise1: matlabshared.tracking.internal.blocks.dialogCallbacksEKFUKFPF(gcbh,'checkboxIsCovarianceTimeVarying','HasTimeVaryingMeasurementNoise1','MeasurementNoise1')
      mask Callback HasMeasurementJacobianFcn2: matlabshared.tracking.internal.blocks.dialogCallbacksEKFUKFPF(gcbh(),'checkBoxHasJacobianFcn','Measurement','2');
      mask TypeOptions HasAdditiveMeasurementNoise2: shared_tracking:blocks:maskPromptEKFUKFAdditiveNoise | shared_tracking:blocks:maskPromptEKFUKFNonAdditiveNoise
      mask Callback HasTimeVaryingMeasurementNoise2: matlabshared.tracking.internal.blocks.dialogCallbacksEKFUKFPF(gcbh,'checkboxIsCovarianceTimeVarying','HasTimeVaryingMeasurementNoise2','MeasurementNoise2')
      mask Callback HasMeasurementJacobianFcn3: matlabshared.tracking.internal.blocks.dialogCallbacksEKFUKFPF(gcbh(),'checkBoxHasJacobianFcn','Measurement','3');
      mask TypeOptions HasAdditiveMeasurementNoise3: shared_tracking:blocks:maskPromptEKFUKFAdditiveNoise | shared_tracking:blocks:maskPromptEKFUKFNonAdditiveNoise
      mask Callback HasTimeVaryingMeasurementNoise3: matlabshared.tracking.internal.blocks.dialogCallbacksEKFUKFPF(gcbh,'checkboxIsCovarianceTimeVarying','HasTimeVaryingMeasurementNoise3','MeasurementNoise3')
      mask Callback HasMeasurementJacobianFcn4: matlabshared.tracking.internal.blocks.dialogCallbacksEKFUKFPF(gcbh(),'checkBoxHasJacobianFcn','Measurement','4');
      mask TypeOptions HasAdditiveMeasurementNoise4: shared_tracking:blocks:maskPromptEKFUKFAdditiveNoise | shared_tracking:blocks:maskPromptEKFUKFNonAdditiveNoise
      mask Callback HasTimeVaryingMeasurementNoise4: matlabshared.tracking.internal.blocks.dialogCallbacksEKFUKFPF(gcbh,'checkboxIsCovarianceTimeVarying','HasTimeVaryingMeasurementNoise4','MeasurementNoise4')
      mask Callback HasMeasurementJacobianFcn5: matlabshared.tracking.internal.blocks.dialogCallbacksEKFUKFPF(gcbh(),'checkBoxHasJacobianFcn','Measurement','5');
      mask TypeOptions HasAdditiveMeasurementNoise5: shared_tracking:blocks:maskPromptEKFUKFAdditiveNoise | shared_tracking:blocks:maskPromptEKFUKFNonAdditiveNoise
      mask Callback HasTimeVaryingMeasurementNoise5: matlabshared.tracking.internal.blocks.dialogCallbacksEKFUKFPF(gcbh,'checkboxIsCovarianceTimeVarying','HasTimeVaryingMeasurementNoise5','MeasurementNoise5')
      mask Callback EnableMultirate: matlabshared.tracking.internal.blocks.dialogCallbacksEKFUKFPF(gcbh,'checkBoxHasMultirate')
      mask TypeOptions DataType: shared_tracking:blocks:maskPromptDouble | shared_tracking:blocks:maskPromptSingle
      mask Callback NumberOfMeasurements: matlabshared.tracking.internal.blocks.dialogCallbacksEKFUKFPF(gcbh,'editboxNumberOfMeasurements','MeasurementFcn');
      mask DialogControl DescGroupVar Prompt: shared_tracking:blocks:maskPromptEKFTitle
      mask DialogControl TabSystemModel Prompt: shared_tracking:blocks:maskPromptSystemModel
      mask DialogControl GroupStateTransition Prompt: shared_tracking:blocks:maskPromptStateTransition
      mask DialogControl StateTransitionFunctionText Prompt: shared_tracking:blocks:maskPromptFunction
      mask DialogControl HasStateTransitionJacobianFcn Prompt: Jacobian
      mask DialogControl Spacer Prompt: (Add text here)
      mask DialogControl ProcessNoiseText Prompt: shared_tracking:blocks:maskPromptEKFUKFProcessNoise
      mask DialogControl ProcessNoiseCovarianceText Prompt: shared_tracking:blocks:maskPromptCovariance
      mask DialogControl HasTimeVaryingProcessNoise Prompt: Time-varying
      mask DialogControl InitializationContainer Prompt: shared_tracking:blocks:maskPromptInitialization
      mask DialogControl InitialStateText Prompt: shared_tracking:blocks:maskPromptEKFUKFInitialState
      mask DialogControl InitialCovarianceText Prompt: shared_tracking:blocks:maskPromptEKFUKFInitialCovariance
      mask DialogControl GroupMeasurement1 Prompt: shared_tracking:blocks:maskPromptMeasurement1
      mask DialogControl MeasurementFunction1Text Prompt: shared_tracking:blocks:maskPromptFunction
      mask DialogControl HasMeasurementJacobianFcn1 Prompt: Jacobian
      mask DialogControl HasMeasurementEnablePort1 Prompt: Add Enable port
      mask DialogControl MeasurementNoiseText1 Prompt: shared_tracking:blocks:maskPromptEKFUKFMeasurementNoise
      mask DialogControl MeasurementNoiseCovarianceText1 Prompt: shared_tracking:blocks:maskPromptCovariance
      mask DialogControl HasTimeVaryingMeasurementNoise1 Prompt: Time-varying
      mask DialogControl GroupMeasurement2 Prompt: shared_tracking:blocks:maskPromptMeasurement2
      mask DialogControl MeasurementFunction2Text Prompt: shared_tracking:blocks:maskPromptFunction
      mask DialogControl HasMeasurementJacobianFcn2 Prompt: Jacobian
      mask DialogControl HasMeasurementEnablePort2 Prompt: Add Enable port
      mask DialogControl MeasurementNoiseText2 Prompt: shared_tracking:blocks:maskPromptEKFUKFMeasurementNoise
      mask DialogControl MeasurementNoiseCovarianceText2 Prompt: shared_tracking:blocks:maskPromptCovariance
      mask DialogControl HasTimeVaryingMeasurementNoise2 Prompt: Time-varying
      mask DialogControl GroupMeasurement3 Prompt: shared_tracking:blocks:maskPromptMeasurement3
      mask DialogControl MeasurementFunction3Text Prompt: shared_tracking:blocks:maskPromptFunction
      mask DialogControl HasMeasurementJacobianFcn3 Prompt: Jacobian
      mask DialogControl HasMeasurementEnablePort3 Prompt: Add Enable port
      mask DialogControl MeasurementNoiseText3 Prompt: shared_tracking:blocks:maskPromptEKFUKFMeasurementNoise
      mask DialogControl MeasurementNoiseCovarianceText3 Prompt: shared_tracking:blocks:maskPromptCovariance
      mask DialogControl HasTimeVaryingMeasurementNoise3 Prompt: Time-varying
      mask DialogControl GroupMeasurement4 Prompt: shared_tracking:blocks:maskPromptMeasurement4
      mask DialogControl MeasurementFunction4Text Prompt: shared_tracking:blocks:maskPromptFunction
      mask DialogControl HasMeasurementJacobianFcn4 Prompt: Jacobian
      mask DialogControl HasMeasurementEnablePort4 Prompt: Add Enable port
      mask DialogControl MeasurementNoiseText4 Prompt: shared_tracking:blocks:maskPromptEKFUKFMeasurementNoise
      mask DialogControl MeasurementNoiseCovarianceText4 Prompt: shared_tracking:blocks:maskPromptCovariance
      mask DialogControl HasTimeVaryingMeasurementNoise4 Prompt: Time-varying
      mask DialogControl GroupMeasurement5 Prompt: shared_tracking:blocks:maskPromptMeasurement5
      mask DialogControl MeasurementFunction5Text Prompt: shared_tracking:blocks:maskPromptFunction
      mask DialogControl HasMeasurementJacobianFcn5 Prompt: Jacobian
      mask DialogControl HasMeasurementEnablePort5 Prompt: Add Enable port
      mask DialogControl MeasurementNoiseText5 Prompt: shared_tracking:blocks:maskPromptEKFUKFMeasurementNoise
      mask DialogControl MeasurementNoiseCovarianceText5 Prompt: shared_tracking:blocks:maskPromptCovariance
      mask DialogControl HasTimeVaryingMeasurementNoise5 Prompt: Time-varying
      mask DialogControl AddMeasurement Prompt: shared_tracking:blocks:maskPromptAddMeasurement
      mask DialogControl AddMeasurement Callback: matlabshared.tracking.internal.blocks.dialogCallbacksEKFUKFPF(gcbh,'buttonAddMeasurement','MeasurementFcn');
      mask DialogControl Spacer1 Prompt: (Add text here)
      mask DialogControl Spacer2 Prompt: (Add text here)
      mask DialogControl Spacer3 Prompt: (Add text here)
      mask DialogControl RemoveMeasurement Prompt: shared_tracking:blocks:maskPromptRemoveMeasurement
      mask DialogControl RemoveMeasurement Callback: matlabshared.tracking.internal.blocks.dialogCallbacksEKFUKFPF(gcbh,'buttonRemoveMeasurement','MeasurementFcn');
      mask DialogControl TabMultirate Prompt: shared_tracking:blocks:maskPromptEKFUKFMultirate
      mask DialogControl GroupMultirate Prompt: shared_tracking:blocks:maskPromptEKFUKFMultirate
      mask DialogControl EnableMultirate Prompt: Enable multirate operation
      mask DialogControl GroupMultirateSampleTimes Prompt: shared_tracking:blocks:maskPromptSampleTimeNoInheritance
      mask DialogControl StateTransitionFcnSampleTime Prompt: State Transition
      mask DialogControl MeasurementFcn1SampleTime Prompt: Measurement 1
      mask DialogControl MeasurementFcn2SampleTime Prompt: Measurement 2
      mask DialogControl MeasurementFcn3SampleTime Prompt: Measurement 3
      mask DialogControl MeasurementFcn4SampleTime Prompt: Measurement 4
      mask DialogControl MeasurementFcn5SampleTime Prompt: Measurement 5
      mask DialogControl ContainerSettings Prompt: shared_tracking:blocks:maskPromptEKFUKFSettings
      mask DialogControl UseCurrentEstimator Prompt: Use the current measurements to improve state estimates
      mask DialogControl OutputStateCovariance Prompt: Output state estimation error covariance
      mask DialogControl DataType Prompt: Data type:
      mask DialogControl SampleTime Prompt: Sample time:
  Generate state estimation error : Sum  Inputs=-+
  Gyroscope Bias : Scope
  MATLAB Function : MATLAB Function  TreatAsAtomicUnit=on
  Measurement Jacobian : MATLAB Function  TreatAsAtomicUnit=on
  Mux2 : Mux  Inputs=2
  Mux4 : Mux  Inputs=2
  Mux5 : Mux  Inputs=2
  Orientation Error : Scope
  RMS : dspstat3/RMS  run=off  directionMode=Each column  dimension=1  InputProcessing=Columns as channels (frame based)  reset_popup=None
  Radians to Degrees : simulink_extras/Transformations/Radians to Degrees
  Selector3 : Selector  InputPortWidth=7  IndexOptions=Index vector (dialog)  Indices=[1:4]  OutputSizes=1
  Selector4 : Selector  InputPortWidth=7  IndexOptions=Index vector (dialog)  Indices=[5:7]  OutputSizes=1
  State Estimation Error : Scope
  Subtract : Sum  Inputs=||+|-
  Sum : Sum  Inputs=-+|
  Terminator : Terminator
  Z-H(x) innovation : Subsystem
  Zero-Order Hold : ZeroOrderHold  SampleTime=Ts
  Zero-Order Hold1 : ZeroOrderHold  SampleTime=Ts
  gravity vector2 : Constant  Value=[0;0;g]
  local magnetic field in NED2 : Constant  Value=IMU.magBn
  measure xk+1 : MATLAB Function  TreatAsAtomicUnit=on
  BUS_EST : Outport
  wires:
  Bus Selector1/1 -> Zero-Order Hold1/1  "<gyro>"
  Bus Selector3/1 -> [q], Mux5/1  "<q>"
  [Sen] -> Bus Selector/1
  Bus Selector/1 -> Mux2/1  "<acc>"
  Bus Selector/2 -> Mux2/2  "<mag>"
  [U] -> Extended Kalman Filter With Analytical Jacobian/3(MeasurementFcn1Inputs)  "constant refs"
  Zero-Order Hold1/1 -> Extended Kalman Filter With Analytical Jacobian/1(StateTransitionFcnInputs)
  Generate state estimation error/1 -> State Estimation Error/1  "state error"
  Zero-Order Hold/1 -> Extended Kalman Filter With Analytical Jacobian/2(y1)
  Extended Kalman Filter With Analytical Jacobian/1(xhat) -> [x_est], Selector4/1, Selector3/1  "xhat[k|k]"
  Radians to Degrees/1 -> Gyroscope Bias/1  "gyro bias err (deg/s)"
  Subtract/1 -> Radians to Degrees/1
  Constant2/1 -> Subtract/2
  MATLAB Function/1(y) -> Orientation Error/1, RMS/1  "Ori error (deg)"
  ground_truth/1 -> Bus Selector3/1
  sensors/1 -> [Sen]
  [Sen] -> Bus Selector1/1
  Mux2/1 -> [Z]  "z[k]"
  [Z] -> Zero-Order Hold/1  "z[k]"
  gravity vector2/1 -> Mux4/1
  local magnetic field in NED2/1 -> Mux4/2
  Mux4/1 -> [U]
  Selector3/1 -> [q_est]
  Selector4/1 -> [b_est]
  [q] -> MATLAB Function/2(v)
  [q_est] -> MATLAB Function/1(u)
  [x_est] -> Generate state estimation error/1
  Mux5/1 -> [x_true]  "x true"
  Constant1/1 -> Mux5/2
  [x_true] -> Generate state estimation error/2
  Extended Kalman Filter With Analytical Jacobian/2(P) -> [P]  "process Covariance"
  [b_est] -> Subtract/1
  Bus Creator/1 -> BUS_EST/1
  [q_est] -> Bus Creator/1  "q_est"
  [b_est] -> Bus Creator/2, Sum/1  "b_est"
  [Sen] -> Bus Selector2/1
  Bus Selector2/2 -> Bus Creator/5  "<acc>"
  Bus Selector2/4 -> Bus Creator/7  "<mag>"
  Bus Selector2/3 -> Bus Creator/6  "<acc_zero>"
  Bus Selector2/1 -> Sum/2, Bus Creator/4  "<gyro>"
  Sum/1 -> Bus Creator/3  "gyro_est"
  Bus Selector2/5 -> Bus Creator/8  "<alt>"
  [Z] -> Z-H(x) innovation/1(z[k])  "z[k]"
  [h_x] -> Z-H(x) innovation/2(h(x))  "h(t)"
  Z-H(x) innovation/1(innovation) -> Terminator/1  "innovation"
  measure xk+1/1(y) -> [h_x]  "h(x)"
  [U] -> measure xk+1/2(u)  "U_const"
  [x_est] -> measure xk+1/1(x)  "x_est[k]"
  [U] -> Measurement Jacobian/2(u)  "U_const"
  [x_est] -> Measurement Jacobian/1(x)  "x_est[k]"
  Measurement Jacobian/1(H) -> [H]  "H"
  RMS/1 -> Display/1
  [P] -> Z-H(x) innovation/3(P)  "P"
  [H] -> Z-H(x) innovation/4(H)  "H"
  Constant/1 -> Z-H(x) innovation/5(R)  "R"
